simulink model "ModelCurrentState"  (R2024b)
settings: Solver=VariableStepAuto  StartTime=0.0  StopTime=StopTime  MaxStep=0.001  RelTol=1e-3
model workspace: external: MAT-File 3DModelInputs.mat (data not in the file)
undefined symbols (not defined in the file): GripStrength, KillswitchFinalValue, KillswitchInitialValue, KillswitchStepTime, LeftLowerArmLength, PlaneTilt, RightLowerArmLength, UpperTorsoLength, X, Y, Z
libraries: nesl_utility x408, sm_lib x139, matrix_library x11, simulink x1
(part 3 of 14)

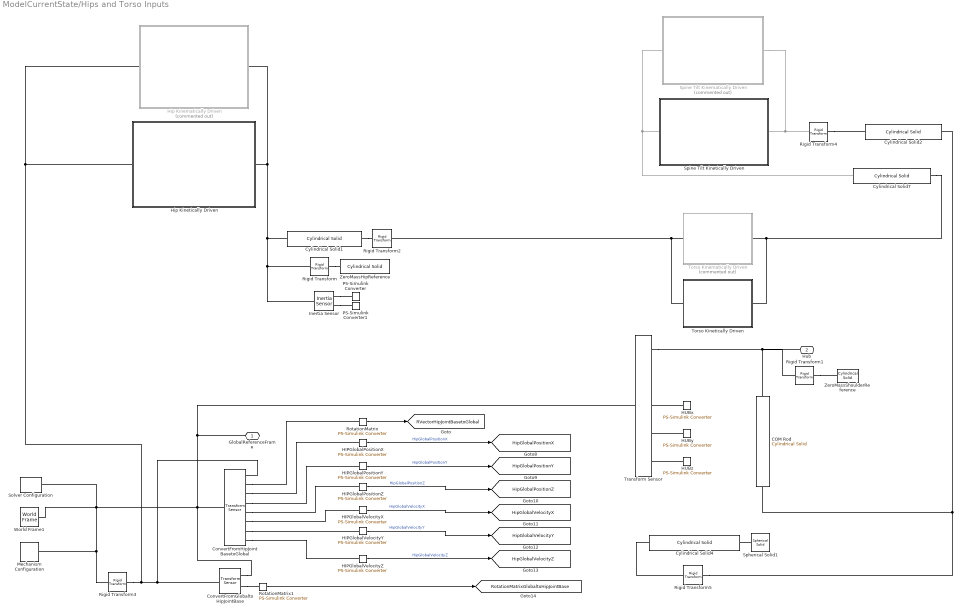
== system ModelCurrentState/Hips and Torso Inputs ==
  COM Rod : sm_lib/Body Elements/Cylindrical Solid  CylinderRadius=0.1  CylinderRadiusUnits=in  CylinderLength=2  CylinderLengthUnits=in  ExportEntireGeometry=off  InertiaType=CalculateFromGeometry  BasedOnType=Mass  Density=1000  DensityUnits=kg/m^3  Mass=0  MassUnits=kg  CenterOfMass=[0 0 0]  CenterOfMassUnits=m  MomentsOfInertia=[1 1 1]  MomentsOfInertiaUnits=kg*m^2  ProductsOfInertia=[0 0 0]  ProductsOfInertiaUnits=kg*m^2  GraphicType=FromGeometry  MarkerShape=Sphere  MarkerSize=10  GraphicVisPropType=SimpleVisualProperties  GraphicDiffuseColor=[0.5 0.5 0.5]  GraphicOpacity=1.0  GraphicSpecularColor=[0.5 0.5 0.5 1.0]  GraphicAmbientColor=[0.15 0.15 0.15 1.0]  GraphicEmissiveColor=[0.0 0.0 0.0 1.0]  GraphicShininess=75  DoExposeReferenceFrame=off  SerializedFrames=<Frames><Frame><Id>Frame1</Id><Value><Name>COM Rod Bottom</Name><Origin><Source>GeometricFeature</Source><FeatureName>top curve</FeatureName></Origin><PrimaryAxis><DefinedDirection>-X</DefinedDirection><Source>ReferenceFrame</Source><SourceDirection>-Y</SourceDirection><FeatureName></FeatureName></PrimaryAxis><SecondaryAxis><DefinedDirection>+Y</DefinedDirection><Source>ReferenceFrame</Source><SourceDirection>+Z</SourceDirection><FeatureName></FeatureName></SecondaryAxis></Value></Frame><Frame><Id>Frame2</Id><Value><Name>COM Rod Top</Name><Origin><Source>GeometricFeature</Source><FeatureName>bottom curve</FeatureName></Origin><PrimaryAxis><DefinedDirection>+X</DefinedDirection><Source>ReferenceFrame</Source><SourceDirection>+X</SourceDirection><FeatureName></FeatureName></PrimaryAxis><SecondaryAxis><DefinedDirection>+Y</DefinedDirection><Source>ReferenceFrame</Source><SourceDirection>+Z</SourceDirection><FeatureName></FeatureName></SecondaryAxis></Value></Frame></Frames>
  ConvertFromGlobaltoHipJointBase : sm_lib/Frames and Transforms/Transform Sensor  MeasurementFrame=World  RotationSequence=XYX  SenseAngle=off  SenseAxis=off  SenseQ=off  SenseR=on  SenseRotationSequence=off  SenseOmegaX=off  SenseOmegaY=off  SenseOmegaZ=off  SenseOmega=off  SenseQDot=off  SenseRDot=off  SenseRotationSequenceDot=off  SenseAlphaX=off  SenseAlphaY=off  SenseAlphaZ=off  SenseAlpha=off  SenseQDDot=off  SenseRDDot=off  SenseX=off  SenseY=off  SenseZ=off  SenseXYZ=off  SenseRad=off  SenseAzim=off  SenseDist=off  SenseInc=off  SenseXDot=off  SenseYDot=off  SenseZDot=off  SenseXYZDot=off  SenseRadDot=off  SenseAzimDot=off  SenseDistDot=off  SenseIncDot=off  SenseXDDot=off  SenseYDDot=off  SenseZDDot=off  SenseXYZDDot=off  SenseRadDDot=off  SenseAzimDDot=off  SenseDistDDot=off  SenseIncDDot=off
  ConvertFromHipJointBasetoGlobal : sm_lib/Frames and Transforms/Transform Sensor  MeasurementFrame=World  RotationSequence=XYX  SenseAngle=off  SenseAxis=off  SenseQ=off  SenseR=on  SenseRotationSequence=off  SenseOmegaX=off  SenseOmegaY=off  SenseOmegaZ=off  SenseOmega=off  SenseQDot=off  SenseRDot=off  SenseRotationSequenceDot=off  SenseAlphaX=off  SenseAlphaY=off  SenseAlphaZ=off  SenseAlpha=off  SenseQDDot=off  SenseRDDot=off  SenseX=on  SenseY=on  SenseZ=on  SenseXYZ=off  SenseRad=off  SenseAzim=off  SenseDist=off  SenseInc=off  SenseXDot=on  SenseYDot=on  SenseZDot=on  SenseXYZDot=off  SenseRadDot=off  SenseAzimDot=off  SenseDistDot=off  SenseIncDot=off  SenseXDDot=off  SenseYDDot=off  SenseZDDot=off  SenseXYZDDot=off  SenseRadDDot=off  SenseAzimDDot=off  SenseDistDDot=off  SenseIncDDot=off
  Cylindrical Solid1 : sm_lib/Body Elements/Cylindrical Solid  CylinderRadius=6  CylinderRadiusUnits=in  CylinderLength=LowerTorsoLength  CylinderLengthUnits=in  ExportEntireGeometry=off  InertiaType=CalculateFromGeometry  BasedOnType=Mass  Density=1000  DensityUnits=kg/m^3  Mass=20  MassUnits=kg  CenterOfMass=[0 0 0]  CenterOfMassUnits=m  MomentsOfInertia=[1 1 1]  MomentsOfInertiaUnits=kg*m^2  ProductsOfInertia=[0 0 0]  ProductsOfInertiaUnits=kg*m^2  GraphicType=FromGeometry  MarkerShape=Sphere  MarkerSize=10  GraphicVisPropType=SimpleVisualProperties  GraphicDiffuseColor=[0.2 0.2 0.0]  GraphicOpacity=1.0  GraphicSpecularColor=[0.5 0.5 0.5 1.0]  GraphicAmbientColor=[0.15 0.15 0.15 1.0]  GraphicEmissiveColor=[0.0 0.0 0.0 1.0]  GraphicShininess=75  DoExposeReferenceFrame=off  SerializedFrames=<Frames><Frame><Id>Frame1</Id><Value><Name>Bottom of Hips</Name><Origin><Source>GeometricFeature</Source><FeatureName>top surface</FeatureName></Origin><PrimaryAxis><DefinedDirection>-Z</DefinedDirection><Source>ReferenceFrame</Source><SourceDirection>+Z</SourceDirection><FeatureName></FeatureName></PrimaryAxis><SecondaryAxis><DefinedDirection>+X</DefinedDirection><Source>ReferenceFrame</Source><SourceDirection>+X</SourceDirection><FeatureName></FeatureName></SecondaryAxis></Value></Frame><Frame><Id>Frame2</Id><Value><Name>Top of Hips</Name><Origin><Source>GeometricFeature</Source><FeatureName>bottom surface</FeatureName></Origin><PrimaryAxis><DefinedDirection>+Z</DefinedDirection><Source>ReferenceFrame</Source><SourceDirection>+Z</SourceDirection><FeatureName></FeatureName></PrimaryAxis><SecondaryAxis><DefinedDirection>+X</DefinedDirection><Source>ReferenceFrame</Source><SourceDirection>+X</SourceDirection><FeatureName></FeatureName></SecondaryAxis></Value></Frame></Frames>
  Cylindrical Solid2 : sm_lib/Body Elements/Cylindrical Solid  CylinderRadius=6  CylinderRadiusUnits=in  CylinderLength=UpperTorsoLength*0.8  CylinderLengthUnits=in  ExportEntireGeometry=off  InertiaType=CalculateFromGeometry  BasedOnType=Mass  Density=1000  DensityUnits=kg/m^3  Mass=20*0.8  MassUnits=kg  CenterOfMass=[0 0 0]  CenterOfMassUnits=m  MomentsOfInertia=[1 1 1]  MomentsOfInertiaUnits=kg*m^2  ProductsOfInertia=[0 0 0]  ProductsOfInertiaUnits=kg*m^2  GraphicType=FromGeometry  MarkerShape=Sphere  MarkerSize=10  GraphicVisPropType=SimpleVisualProperties  GraphicDiffuseColor=[0.2 0.2 1.0]  GraphicOpacity=1.0  GraphicSpecularColor=[0.5 0.5 0.5 1.0]  GraphicAmbientColor=[0.15 0.15 0.15 1.0]  GraphicEmissiveColor=[0.0 0.0 0.0 1.0]  GraphicShininess=75  DoExposeReferenceFrame=off  SerializedFrames=<Frames><Frame><Id>Frame1</Id><Value><Name>Bottom of Torso</Name><Origin><Source>GeometricFeature</Source><FeatureName>top surface</FeatureName></Origin><PrimaryAxis><DefinedDirection>-Z</DefinedDirection><Source>ReferenceFrame</Source><SourceDirection>+Z</SourceDirection><FeatureName></FeatureName></PrimaryAxis><SecondaryAxis><DefinedDirection>+X</DefinedDirection><Source>ReferenceFrame</Source><SourceDirection>+X</SourceDirection><FeatureName></FeatureName></SecondaryAxis></Value></Frame><Frame><Id>Frame2</Id><Value><Name>Top of Torso</Name><Origin><Source>GeometricFeature</Source><FeatureName>bottom surface</FeatureName></Origin><PrimaryAxis><DefinedDirection>+Z</DefinedDirection><Source>ReferenceFrame</Source><SourceDirection>+Z</SourceDirection><FeatureName></FeatureName></PrimaryAxis><SecondaryAxis><DefinedDirection>+X</DefinedDirection><Source>ReferenceFrame</Source><SourceDirection>+X</SourceDirection><FeatureName></FeatureName></SecondaryAxis></Value></Frame></Frames>
  Cylindrical Solid4 : sm_lib/Body Elements/Cylindrical Solid  CylinderRadius=2  CylinderRadiusUnits=in  CylinderLength=10  CylinderLengthUnits=in  ExportEntireGeometry=off  InertiaType=CalculateFromGeometry  BasedOnType=Density  Density=1000  DensityUnits=kg/m^3  Mass=1  MassUnits=kg  CenterOfMass=[0 0 0]  CenterOfMassUnits=m  MomentsOfInertia=[1 1 1]  MomentsOfInertiaUnits=kg*m^2  ProductsOfInertia=[0 0 0]  ProductsOfInertiaUnits=kg*m^2  GraphicType=FromGeometry  MarkerShape=Sphere  MarkerSize=10  GraphicVisPropType=SimpleVisualProperties  GraphicDiffuseColor=[1.0 0.8 0.4]  GraphicOpacity=1.0  GraphicSpecularColor=[0.5 0.5 0.5 1.0]  GraphicAmbientColor=[0.15 0.15 0.15 1.0]  GraphicEmissiveColor=[0.0 0.0 0.0 1.0]  GraphicShininess=75  DoExposeReferenceFrame=off  SerializedFrames=<Frames><Frame><Id>Frame1</Id><Value><Name>Bottom of Neck</Name><Origin><Source>GeometricFeature</Source><FeatureName>top surface</FeatureName></Origin><PrimaryAxis><DefinedDirection>+Z</DefinedDirection><Source>ReferenceFrame</Source><SourceDirection>+Z</SourceDirection><FeatureName></FeatureName></PrimaryAxis><SecondaryAxis><DefinedDirection>+X</DefinedDirection><Source>ReferenceFrame</Source><SourceDirection>+X</SourceDirection><FeatureName></FeatureName></SecondaryAxis></Value></Frame><Frame><Id>Frame2</Id><Value><Name>Top of Neck</Name><Origin><Source>GeometricFeature</Source><FeatureName>bottom surface</FeatureName></Origin><PrimaryAxis><DefinedDirection>+Z</DefinedDirection><Source>ReferenceFrame</Source><SourceDirection>+Z</SourceDirection><FeatureName></FeatureName></PrimaryAxis><SecondaryAxis><DefinedDirection>+X</DefinedDirection><Source>ReferenceFrame</Source><SourceDirection>+X</SourceDirection><FeatureName></FeatureName></SecondaryAxis></Value></Frame></Frames>
  Cylindrical Solid7 : sm_lib/Body Elements/Cylindrical Solid  CylinderRadius=6  CylinderRadiusUnits=in  CylinderLength=UpperTorsoLength*0.2  CylinderLengthUnits=in  ExportEntireGeometry=off  InertiaType=CalculateFromGeometry  BasedOnType=Mass  Density=1000  DensityUnits=kg/m^3  Mass=20*0.2  MassUnits=kg  CenterOfMass=[0 0 0]  CenterOfMassUnits=m  MomentsOfInertia=[1 1 1]  MomentsOfInertiaUnits=kg*m^2  ProductsOfInertia=[0 0 0]  ProductsOfInertiaUnits=kg*m^2  GraphicType=FromGeometry  MarkerShape=Sphere  MarkerSize=10  GraphicVisPropType=SimpleVisualProperties  GraphicDiffuseColor=[0.2 0.2 1.0]  GraphicOpacity=1.0  GraphicSpecularColor=[0.5 0.5 0.5 1.0]  GraphicAmbientColor=[0.15 0.15 0.15 1.0]  GraphicEmissiveColor=[0.0 0.0 0.0 1.0]  GraphicShininess=75  DoExposeReferenceFrame=off  SerializedFrames=<Frames><Frame><Id>Frame1</Id><Value><Name>Bottom of Torso</Name><Origin><Source>GeometricFeature</Source><FeatureName>top surface</FeatureName></Origin><PrimaryAxis><DefinedDirection>-Z</DefinedDirection><Source>ReferenceFrame</Source><SourceDirection>+Z</SourceDirection><FeatureName></FeatureName></PrimaryAxis><SecondaryAxis><DefinedDirection>+X</DefinedDirection><Source>ReferenceFrame</Source><SourceDirection>+X</SourceDirection><FeatureName></FeatureName></SecondaryAxis></Value></Frame><Frame><Id>Frame2</Id><Value><Name>Top of Torso</Name><Origin><Source>GeometricFeature</Source><FeatureName>bottom surface</FeatureName></Origin><PrimaryAxis><DefinedDirection>+Z</DefinedDirection><Source>ReferenceFrame</Source><SourceDirection>+Z</SourceDirection><FeatureName></FeatureName></PrimaryAxis><SecondaryAxis><DefinedDirection>+X</DefinedDirection><Source>ReferenceFrame</Source><SourceDirection>+X</SourceDirection><FeatureName></FeatureName></SecondaryAxis></Value></Frame></Frames>
  HIPGlobalPositionX : nesl_utility/PS-Simulink Converter  PhysicalDomain=network_engine_domain  SubClassName=ps_output  LeftPortType=input  RightPortType=output  PseudoPeriodic=off  Frequencies=[]  VectorFormat=inherit  Unit=m  AffineConversion=off
  HIPGlobalPositionY : nesl_utility/PS-Simulink Converter  PhysicalDomain=network_engine_domain  SubClassName=ps_output  LeftPortType=input  RightPortType=output  PseudoPeriodic=off  Frequencies=[]  VectorFormat=inherit  Unit=m  AffineConversion=off
  HIPGlobalPositionZ : nesl_utility/PS-Simulink Converter  PhysicalDomain=network_engine_domain  SubClassName=ps_output  LeftPortType=input  RightPortType=output  PseudoPeriodic=off  Frequencies=[]  VectorFormat=inherit  Unit=m  AffineConversion=off
  HIPGlobalVelocityX : nesl_utility/PS-Simulink Converter  PhysicalDomain=network_engine_domain  SubClassName=ps_output  LeftPortType=input  RightPortType=output  PseudoPeriodic=off  Frequencies=[]  VectorFormat=1-D array  Unit=m/s  AffineConversion=off
  HIPGlobalVelocityY : nesl_utility/PS-Simulink Converter  PhysicalDomain=network_engine_domain  SubClassName=ps_output  LeftPortType=input  RightPortType=output  PseudoPeriodic=off  Frequencies=[]  VectorFormat=1-D array  Unit=m/s  AffineConversion=off
  HIPGlobalVelocityZ : nesl_utility/PS-Simulink Converter  PhysicalDomain=network_engine_domain  SubClassName=ps_output  LeftPortType=input  RightPortType=output  PseudoPeriodic=off  Frequencies=[]  VectorFormat=1-D array  Unit=m/s  AffineConversion=off
  HUBx : nesl_utility/PS-Simulink Converter  PhysicalDomain=network_engine_domain  SubClassName=ps_output  LeftPortType=input  RightPortType=output  PseudoPeriodic=off  Frequencies=[]  VectorFormat=1-D array  Unit=inherit  AffineConversion=off
  HUBy : nesl_utility/PS-Simulink Converter  PhysicalDomain=network_engine_domain  SubClassName=ps_output  LeftPortType=input  RightPortType=output  PseudoPeriodic=off  Frequencies=[]  VectorFormat=1-D array  Unit=inherit  AffineConversion=off
  HUBz : nesl_utility/PS-Simulink Converter  PhysicalDomain=network_engine_domain  SubClassName=ps_output  LeftPortType=input  RightPortType=output  PseudoPeriodic=off  Frequencies=[]  VectorFormat=1-D array  Unit=inherit  AffineConversion=off
  Hip Kinematically Driven : Subsystem  Commented=on
  Hip Kinetically Driven : Subsystem
  Inertia Sensor : sm_lib/Body Elements/Inertia Sensor  SensorExtent=Mechanism  SpanWeldJoints=off  ExcludeGroundedBodies=off  MeasurementFrame=World  SenseMass=on  SenseCenterOfMass=on  SenseInertiaMatrix=off  SenseCenteredInertiaMatrix=off  SensePrincipalInertiaMatrix=off  SenseRotationMatrix=off  GraphicType=None  PrincipalInertiaFrameSize=20  GraphicVisPropType=SimpleVisualProperties  GraphicDiffuseColor=[0.5 0.5 0.5]  GraphicOpacity=1  GraphicSpecularColor=[0.5 0.5 0.5 1.0]  GraphicAmbientColor=[0.15 0.15 0.15 1.0]  GraphicEmissiveColor=[0.0 0.0 0.0 1.0]  GraphicShininess=75
  Mechanism Configuration : sm_lib/Utilities/Mechanism Configuration  UniformGravity=Constant  GravityVector=[0 0 -9.80665]  GravityVectorUnits=m/s^2  LinearizationDelta=0.001  JointModeTransitionNonlinearIterations=2
  PS-Simulink Converter : nesl_utility/PS-Simulink Converter  PhysicalDomain=network_engine_domain  SubClassName=ps_output  LeftPortType=input  RightPortType=output  PseudoPeriodic=off  Frequencies=[]  VectorFormat=1-D array  Unit=inherit  AffineConversion=off
  PS-Simulink Converter1 : nesl_utility/PS-Simulink Converter  PhysicalDomain=network_engine_domain  SubClassName=ps_output  LeftPortType=input  RightPortType=output  PseudoPeriodic=off  Frequencies=[]  VectorFormat=1-D array  Unit=inherit  AffineConversion=off
  Rigid Transform : sm_lib/Frames and Transforms/Rigid Transform  RotationMethod=RotationSequence  FollAlignAxisA=+X  BaseAlignAxisA=+Y  FollAlignAxisB=+Y  BaseAlignAxisB=+Z  RotationStandardAxis=+Z  RotationAngle=0.0  RotationAngleUnits=deg  RotationArbitraryAxis=[0 0 1]  RotationSequenceAxes=BaseAxes  RotationSequence=XYX  RotationSequenceAngles=[0 90 0]  RotationSequenceAnglesUnits=deg  RotationMatrix=[1 0 0; 0 1 0; 0 0 1]  Quaternion=[1 0 0 0]  TranslationMethod=None  TranslationCartesianOffset=[0 0 0]  TranslationCartesianOffsetUnits=m  TranslationStandardAxis=+Z  TranslationStandardOffset=0  TranslationStandardOffsetUnits=m  TranslationROffset=0  TranslationROffsetUnits=m  TranslationThetaOffset=0  TranslationThetaOffsetUnits=deg  TranslationZOffset=0  TranslationZOffsetUnits=m
  Rigid Transform1 : sm_lib/Frames and Transforms/Rigid Transform  RotationMethod=RotationSequence  FollAlignAxisA=+X  BaseAlignAxisA=+Y  FollAlignAxisB=+Y  BaseAlignAxisB=+Z  RotationStandardAxis=+Z  RotationAngle=0.0  RotationAngleUnits=deg  RotationArbitraryAxis=[0 0 1]  RotationSequenceAxes=BaseAxes  RotationSequence=XYX  RotationSequenceAngles=[0 0 0]  RotationSequenceAnglesUnits=deg  RotationMatrix=[1 0 0; 0 1 0; 0 0 1]  Quaternion=[1 0 0 0]  TranslationMethod=None  TranslationCartesianOffset=[0 0 0]  TranslationCartesianOffsetUnits=m  TranslationStandardAxis=+Z  TranslationStandardOffset=0  TranslationStandardOffsetUnits=m  TranslationROffset=0  TranslationROffsetUnits=m  TranslationThetaOffset=0  TranslationThetaOffsetUnits=deg  TranslationZOffset=0  TranslationZOffsetUnits=m
  Rigid Transform2 : sm_lib/Frames and Transforms/Rigid Transform  RotationMethod=RotationSequence  FollAlignAxisA=+X  BaseAlignAxisA=+Y  FollAlignAxisB=+Y  BaseAlignAxisB=+Z  RotationStandardAxis=+Z  RotationAngle=0.0  RotationAngleUnits=deg  RotationArbitraryAxis=[0 0 1]  RotationSequenceAxes=BaseAxes  RotationSequence=XYZ  RotationSequenceAngles=[180 0 0]  RotationSequenceAnglesUnits=deg  RotationMatrix=[1 0 0; 0 1 0; 0 0 1]  Quaternion=[1 0 0 0]  TranslationMethod=None  TranslationCartesianOffset=[0 0 0]  TranslationCartesianOffsetUnits=m  TranslationStandardAxis=+Z  TranslationStandardOffset=0  TranslationStandardOffsetUnits=m  TranslationROffset=0  TranslationROffsetUnits=m  TranslationThetaOffset=0  TranslationThetaOffsetUnits=deg  TranslationZOffset=0  TranslationZOffsetUnits=m
  Rigid Transform3 : sm_lib/Frames and Transforms/Rigid Transform  RotationMethod=RotationSequence  FollAlignAxisA=+X  BaseAlignAxisA=+Y  FollAlignAxisB=+Y  BaseAlignAxisB=+Z  RotationStandardAxis=+Z  RotationAngle=0.0  RotationAngleUnits=deg  RotationArbitraryAxis=[0 0 1]  RotationSequenceAxes=BaseAxes  RotationSequence=ZXZ  RotationSequenceAngles=[0 PlaneTilt 0]  RotationSequenceAnglesUnits=deg  RotationMatrix=[1 0 0; 0 1 0; 0 0 1]  Quaternion=[1 0 0 0]  TranslationMethod=None  TranslationCartesianOffset=[0 0 0]  TranslationCartesianOffsetUnits=m  TranslationStandardAxis=+Z  TranslationStandardOffset=0  TranslationStandardOffsetUnits=m  TranslationROffset=0  TranslationROffsetUnits=m  TranslationThetaOffset=0  TranslationThetaOffsetUnits=deg  TranslationZOffset=0  TranslationZOffsetUnits=m
  Rigid Transform4 : sm_lib/Frames and Transforms/Rigid Transform  RotationMethod=RotationSequence  FollAlignAxisA=+X  BaseAlignAxisA=+Y  FollAlignAxisB=+Y  BaseAlignAxisB=+Z  RotationStandardAxis=+Z  RotationAngle=0  RotationAngleUnits=deg  RotationArbitraryAxis=[0 0 1]  RotationSequenceAxes=FollowerAxes  RotationSequence=XYZ  RotationSequenceAngles=[180 0 0]  RotationSequenceAnglesUnits=deg  RotationMatrix=[1 0 0;0 1 0;0 0 1]  Quaternion=[1 0 0 0]  TranslationMethod=None  TranslationCartesianOffset=[0 0 0]  TranslationCartesianOffsetUnits=m  TranslationStandardAxis=+Z  TranslationStandardOffset=0  TranslationStandardOffsetUnits=m  TranslationROffset=0  TranslationROffsetUnits=m  TranslationThetaOffset=0  TranslationThetaOffsetUnits=deg  TranslationZOffset=0  TranslationZOffsetUnits=m
  Rigid Transform5 : sm_lib/Frames and Transforms/Rigid Transform  RotationMethod=RotationSequence  FollAlignAxisA=+X  BaseAlignAxisA=+Y  FollAlignAxisB=+Y  BaseAlignAxisB=+Z  RotationStandardAxis=+Z  RotationAngle=0.0  RotationAngleUnits=deg  RotationArbitraryAxis=[0 0 1]  RotationSequenceAxes=BaseAxes  RotationSequence=XYX  RotationSequenceAngles=[0 0 0]  RotationSequenceAnglesUnits=deg  RotationMatrix=[1 0 0; 0 1 0; 0 0 1]  Quaternion=[1 0 0 0]  TranslationMethod=None  TranslationCartesianOffset=[0 0 0]  TranslationCartesianOffsetUnits=m  TranslationStandardAxis=+Z  TranslationStandardOffset=0  TranslationStandardOffsetUnits=m  TranslationROffset=0  TranslationROffsetUnits=m  TranslationThetaOffset=0  TranslationThetaOffsetUnits=deg  TranslationZOffset=0  TranslationZOffsetUnits=m
  RotationMatrix : nesl_utility/PS-Simulink Converter  PhysicalDomain=network_engine_domain  SubClassName=ps_output  LeftPortType=input  RightPortType=output  PseudoPeriodic=off  Frequencies=[]  VectorFormat=1-D array  Unit=inherit  AffineConversion=off
  RotationMatrix1 : nesl_utility/PS-Simulink Converter  PhysicalDomain=network_engine_domain  SubClassName=ps_output  LeftPortType=input  RightPortType=output  PseudoPeriodic=off  Frequencies=[]  VectorFormat=1-D array  Unit=inherit  AffineConversion=off
  Solver Configuration : nesl_utility/Solver Configuration  PhysicalDomain=network_engine_domain  SubClassName=solver  LeftPortType=input  RightPortType=generic  Tones=[]  Harmonics=[]  SimulateNoise=off  Profile=off  UseLocalSampling=off  EnableSwitchedLinearOptims=on  FrequencyDomain=off  UseCCode=off  RelTol=0.001  AbsTol=0.001  MinStep=1e-09  ToWorkspace=off  RevertToSquareIcSolve=off  NumHomotopyIterations=100  PhasorMode=off  PhasorModeNumHarmonics=1  ConsistencySolver=NEWTON_XTOL_AFTER_FTOL  IndexReductionMethod=DerivativeReplacement  DoDC=off  ResidualTolerance=1e-09  ConsistencyTolSource=GLOBAL  ConsistencyAbsTol=0.001  ConsistencyRelTol=0.001  ConsistencyTolFactor=0.001  UseLocalSolver=off  LocalSolverChoice=NE_BACKWARD_EULER_ADVANCER  ResolveIndetEquations=on  FunctionEvalNumThread=1  LocalSolverSampleTime=0.001  DoFixedCost=off  MaxNonlinIter=3  MaxModeIter=2  ComputeImpulses=off  ImpulseIterations=2  LinearAlgebra=auto  LinearAlgebraNumThread=0  EquationFormulation=NE_TIME_EF  DelaysMemoryBudget=1024  AutomaticFiltering=on  FilteringTimeConstant=0.001  PartitionStorageMethod=AS_NEEDED  PartitionMemoryBudget=1024  PartitionMethod=ROBUST  MultibodyUseLocalSolver=off  MultibodyLocalSolverChoice=ODE1  MultibodyLocalSolverSampleTime=0.001
  Spherical Solid1 : sm_lib/Body Elements/Spherical Solid  SphereRadius=5  SphereRadiusUnits=in  ExportEntireGeometry=off  InertiaType=CalculateFromGeometry  BasedOnType=Mass  Density=1000  DensityUnits=kg/m^3  Mass=11  MassUnits=lbm  CenterOfMass=[0 0 0]  CenterOfMassUnits=m  MomentsOfInertia=[1 1 1]  MomentsOfInertiaUnits=kg*m^2  ProductsOfInertia=[0 0 0]  ProductsOfInertiaUnits=kg*m^2  GraphicType=FromGeometry  MarkerShape=Sphere  MarkerSize=10  GraphicVisPropType=SimpleVisualProperties  GraphicDiffuseColor=[1.0 0.8 0.4]  GraphicOpacity=1.0  GraphicSpecularColor=[0.5 0.5 0.5 1.0]  GraphicAmbientColor=[0.15 0.15 0.15 1.0]  GraphicEmissiveColor=[0.0 0.0 0.0 1.0]  GraphicShininess=75  DoExposeReferenceFrame=on  SerializedFrames=<Frames/>
  Spine Tilt Kinematically Driven : Subsystem  Commented=on
  Spine Tilt Kinetically Driven : Subsystem
  Torso Kinematically Driven : Subsystem  Commented=on
  Torso Kinetically Driven : Subsystem
  Transform Sensor : sm_lib/Frames and Transforms/Transform Sensor  MeasurementFrame=World  RotationSequence=XYX  SenseAngle=off  SenseAxis=off  SenseQ=off  SenseR=on  SenseRotationSequence=off  SenseOmegaX=off  SenseOmegaY=off  SenseOmegaZ=off  SenseOmega=off  SenseQDot=off  SenseRDot=off  SenseRotationSequenceDot=off  SenseAlphaX=off  SenseAlphaY=off  SenseAlphaZ=off  SenseAlpha=off  SenseQDDot=off  SenseRDDot=off  SenseX=on  SenseY=on  SenseZ=on  SenseXYZ=off  SenseRad=off  SenseAzim=off  SenseDist=off  SenseInc=off  SenseXDot=off  SenseYDot=off  SenseZDot=off  SenseXYZDot=off  SenseRadDot=off  SenseAzimDot=off  SenseDistDot=off  SenseIncDot=off  SenseXDDot=off  SenseYDDot=off  SenseZDDot=off  SenseXYZDDot=off  SenseRadDDot=off  SenseAzimDDot=off  SenseDistDDot=off  SenseIncDDot=off
  World Frame1 : sm_lib/Frames and Transforms/World Frame
  ZeroMassHipReference : sm_lib/Body Elements/Cylindrical Solid  CylinderRadius=4  CylinderRadiusUnits=in  CylinderLength=12  CylinderLengthUnits=in  ExportEntireGeometry=off  InertiaType=CalculateFromGeometry  BasedOnType=Mass  Density=1000  DensityUnits=kg/m^3  Mass=0  MassUnits=kg  CenterOfMass=[0 0 0]  CenterOfMassUnits=m  MomentsOfInertia=[1 1 1]  MomentsOfInertiaUnits=kg*m^2  ProductsOfInertia=[0 0 0]  ProductsOfInertiaUnits=kg*m^2  GraphicType=FromGeometry  MarkerShape=Sphere  MarkerSize=10  GraphicVisPropType=SimpleVisualProperties  GraphicDiffuseColor=[0.2 0.2 0.0]  GraphicOpacity=1.0  GraphicSpecularColor=[0.5 0.5 0.5 1.0]  GraphicAmbientColor=[0.15 0.15 0.15 1.0]  GraphicEmissiveColor=[0.0 0.0 0.0 1.0]  GraphicShininess=75  DoExposeReferenceFrame=on  SerializedFrames=<Frames/>
  ZeroMassShoulderReference : sm_lib/Body Elements/Cylindrical Solid  CylinderRadius=3  CylinderRadiusUnits=in  CylinderLength=12  CylinderLengthUnits=in  ExportEntireGeometry=off  InertiaType=CalculateFromGeometry  BasedOnType=Mass  Density=1000  DensityUnits=kg/m^3  Mass=0  MassUnits=kg  CenterOfMass=[0 0 0]  CenterOfMassUnits=m  MomentsOfInertia=[1 1 1]  MomentsOfInertiaUnits=kg*m^2  ProductsOfInertia=[0 0 0]  ProductsOfInertiaUnits=kg*m^2  GraphicType=FromGeometry  MarkerShape=Sphere  MarkerSize=10  GraphicVisPropType=SimpleVisualProperties  GraphicDiffuseColor=[0.07451 0.6235 1]  GraphicOpacity=1.0  GraphicSpecularColor=[0.5 0.5 0.5 1.0]  GraphicAmbientColor=[0.15 0.15 0.15 1.0]  GraphicEmissiveColor=[0.0 0.0 0.0 1.0]  GraphicShininess=75  DoExposeReferenceFrame=on  SerializedFrames=<Frames/>
  GlobalReferenceFrame : PMIOPort  Side=Right
  Hub : PMIOPort  Port=2  Side=Left
  tag scope: HipGlobalPositionX=global, HipGlobalPositionY=global, HipGlobalPositionZ=global, HipGlobalVelocityX=global, HipGlobalVelocityY=global, HipGlobalVelocityZ=global, RVectorHipJointBasetoGlobal=global, RotationMatrixGlobaltoHipJointBase=global
  wires:
  RotationMatrix1/1 -> [RotationMatrixGlobaltoHipJointBase]
  HIPGlobalVelocityZ/1 -> [HipGlobalVelocityZ]  "HipGlobalVelocityZ"
  HIPGlobalVelocityY/1 -> [HipGlobalVelocityY]  "HipGlobalVelocityY"
  HIPGlobalVelocityX/1 -> [HipGlobalVelocityX]  "HipGlobalVelocityX"
  HIPGlobalPositionY/1 -> [HipGlobalPositionY]  "HipGlobalPositionY"
  HIPGlobalPositionX/1 -> [HipGlobalPositionX]  "HipGlobalPositionX"
  HIPGlobalPositionZ/1 -> [HipGlobalPositionZ]  "HipGlobalPositionZ"
  RotationMatrix/1 -> [RVectorHipJointBasetoGlobal]
  connections:
  HUBy/LConn1 -- Transform Sensor/RConn4
  Spine Tilt Kinematically Driven/LConn1 -- Cylindrical Solid7/RConn1 -- Spine Tilt Kinetically Driven/LConn1
  COM Rod/RConn1 -- Transform Sensor/RConn1 -- Rigid Transform1/RConn1 -- Hub/RConn1
  Rigid Transform5/LConn1 -- COM Rod/LConn1 -- Cylindrical Solid2/RConn1
  Rigid Transform1/LConn1 -- ZeroMassShoulderReference/RConn1
  HUBx/LConn1 -- Transform Sensor/RConn3
  Spherical Solid1/RConn1 -- Cylindrical Solid4/RConn1
  Rigid Transform5/RConn1 -- Cylindrical Solid4/LConn1
  HUBz/LConn1 -- Transform Sensor/RConn5
  Rigid Transform4/RConn1 -- Cylindrical Solid2/LConn1
  Transform Sensor/LConn1 -- GlobalReferenceFrame/RConn1 -- ConvertFromHipJointBasetoGlobal/LConn1 -- ConvertFromGlobaltoHipJointBase/RConn1 -- Solver Configuration/RConn1 -- Mechanism Configuration/RConn1 -- Rigid Transform3/LConn1 -- World Frame1/RConn1
  ConvertFromGlobaltoHipJointBase/RConn2 -- RotationMatrix1/LConn1
  ConvertFromHipJointBasetoGlobal/RConn8 -- HIPGlobalVelocityZ/LConn1
  ConvertFromHipJointBasetoGlobal/RConn7 -- HIPGlobalVelocityY/LConn1
  ConvertFromHipJointBasetoGlobal/RConn6 -- HIPGlobalVelocityX/LConn1
  ConvertFromHipJointBasetoGlobal/RConn3 -- HIPGlobalPositionX/LConn1
  Rigid Transform/LConn1 -- ZeroMassHipReference/RConn1
  ConvertFromHipJointBasetoGlobal/RConn4 -- HIPGlobalPositionY/LConn1
  Inertia Sensor/RConn2 -- PS-Simulink Converter1/LConn1
  Inertia Sensor/RConn1 -- PS-Simulink Converter/LConn1
  Cylindrical Solid1/RConn1 -- Rigid Transform2/LConn1
  ConvertFromHipJointBasetoGlobal/RConn2 -- RotationMatrix/LConn1
  ConvertFromHipJointBasetoGlobal/RConn5 -- HIPGlobalPositionZ/LConn1
  Cylindrical Solid7/LConn1 -- Torso Kinetically Driven/RConn1 -- Torso Kinematically Driven/RConn1
  Cylindrical Solid1/LConn1 -- Inertia Sensor/LConn1 -- Rigid Transform/RConn1 -- Hip Kinetically Driven/RConn1 -- Hip Kinematically Driven/RConn1
  Rigid Transform3/RConn1 -- ConvertFromGlobaltoHipJointBase/LConn1 -- ConvertFromHipJointBasetoGlobal/RConn1 -- Hip Kinetically Driven/LConn1 -- Hip Kinematically Driven/LConn1
  Spine Tilt Kinematically Driven/RConn1 -- Rigid Transform4/LConn1 -- Spine Tilt Kinetically Driven/RConn1
  Torso Kinetically Driven/LConn1 -- Rigid Transform2/RConn1 -- Torso Kinematically Driven/LConn1

== system ModelCurrentState/LE Input Function ==
  Left Elbow Input Torque : MATLAB Function  TreatAsAtomicUnit=on  SystemSampleTime=0
  tag scope: FcnOutLEAcceleration=global, FcnOutLEPosition=global, FcnOutLETorque=global, FcnOutLEVelocity=global
  wires:
  [LEPosition] -> Left Elbow Input Torque/3(LEPosition)
  [Time] -> Left Elbow Input Torque/1(Time)
  [LEVelocity] -> Left Elbow Input Torque/4(LEVelocity)
  Left Elbow Input Torque/2(LEPositionInput) -> [FcnOutLEPosition]
  Left Elbow Input Torque/1(JointTorqueLE) -> [FcnOutLETorque]  "LETorqueInput"
  Left Elbow Input Torque/3(LEVelocityInput) -> [FcnOutLEVelocity]
  [Killswitch] -> Left Elbow Input Torque/2(Killswitch)
  Left Elbow Input Torque/4(LEAccelerationInput) -> [FcnOutLEAcceleration]

== system ModelCurrentState/LF Input Function ==
  LF Input Torque : MATLAB Function  TreatAsAtomicUnit=on  SystemSampleTime=0
  tag scope: FcnOutLFAcceleration=global, FcnOutLFPosition=global, FcnOutLFTorque=global, FcnOutLFVelocity=global
  wires:
  LF Input Torque/3(LFVelocityInput) -> [FcnOutLFVelocity]
  LF Input Torque/2(LFPositionInput) -> [FcnOutLFPosition]
  [Killswitch] -> LF Input Torque/2(Killswitch)
  [LFPosition] -> LF Input Torque/3(LFPosition)
  [LFVelocity] -> LF Input Torque/4(LFVelocity)
  [Time] -> LF Input Torque/1(Time)
  LF Input Torque/1(JointTorqueLF) -> [FcnOutLFTorque]  "LFTorqueInput"
  LF Input Torque/4(LFAccelerationInput) -> [FcnOutLFAcceleration]

== system ModelCurrentState/LS Input Function ==
  Left Shoulder Torque Output : MATLAB Function  TreatAsAtomicUnit=on  SystemSampleTime=0
  tag scope: FcnOutLSAccelerationX=global, FcnOutLSAccelerationY=global, FcnOutLSAccelerationZ=global, FcnOutLSPositionX=global, FcnOutLSPositionY=global, FcnOutLSPositionZ=global, FcnOutLSTorqueX=global, FcnOutLSTorqueY=global, FcnOutLSTorqueZ=global, FcnOutLSVelocityX=global, FcnOutLSVelocityY=global, FcnOutLSVelocityZ=global
  wires:
  [Killswitch] -> Left Shoulder Torque Output/2(Killswitch)
  Left Shoulder Torque Output/1(JointTorqueLSX) -> [FcnOutLSTorqueX]  "LSTorqueXInput"
  Left Shoulder Torque Output/4(LSPositionInputX) -> [FcnOutLSPositionX]  "LSPositionX"
  Left Shoulder Torque Output/7(LSVelocityInputX) -> [FcnOutLSVelocityX]  "LSVelocityX"
  [Time] -> Left Shoulder Torque Output/1(Time)
  Left Shoulder Torque Output/12(LSAccelerationInputZ) -> [FcnOutLSAccelerationZ]  "LSAccelerationZ"
  Left Shoulder Torque Output/2(JointTorqueLSY) -> [FcnOutLSTorqueY]  "LSTorqueYInput"
  Left Shoulder Torque Output/8(LSVelocityInputY) -> [FcnOutLSVelocityY]  "LSVelocityY"
  Left Shoulder Torque Output/11(LSAccelerationInputY) -> [FcnOutLSAccelerationY]  "LSAccelerationY"
  Left Shoulder Torque Output/5(LSPositionInputY) -> [FcnOutLSPositionY]  "LSPositionY"
  Left Shoulder Torque Output/10(LSAccelerationInputX) -> [FcnOutLSAccelerationX]  "LSAccelerationX"
  Left Shoulder Torque Output/9(LSVelocityInputZ) -> [FcnOutLSVelocityZ]  "LSVelocityZ"
  Left Shoulder Torque Output/3(JointTorqueLSZ) -> [FcnOutLSTorqueZ]  "LSTorqueZInput"
  Left Shoulder Torque Output/6(LSPositionInputZ) -> [FcnOutLSPositionZ]  "LSPositionZ"
  [LSPositionX] -> Left Shoulder Torque Output/3(LSPositionX)
  [LSPositionY] -> Left Shoulder Torque Output/4(LSPositionY)
  [LSPositionZ] -> Left Shoulder Torque Output/5(LSPositionZ)
  [LSVelocityX] -> Left Shoulder Torque Output/6(LSVelocityX)
  [LSVelocityY] -> Left Shoulder Torque Output/7(LSVelocityY)
  [LSVelocityZ] -> Left Shoulder Torque Output/8(LSVelocityZ)

== system ModelCurrentState/LScap Input Function ==
  LScap Torque : MATLAB Function  TreatAsAtomicUnit=on  SystemSampleTime=0
  tag scope: FcnOutLScapAccelerationX=global, FcnOutLScapAccelerationY=global, FcnOutLScapPositionX=global, FcnOutLScapPositionY=global, FcnOutLScapTorqueX=global, FcnOutLScapTorqueY=global, FcnOutLScapVelocityX=global, FcnOutLScapVelocityY=global
  wires:
  LScap Torque/1(JointTorqueLScapX) -> [FcnOutLScapTorqueX]  "LScapTorqueXInput"
  LScap Torque/6(LScapVelocityInputY) -> [FcnOutLScapVelocityY]
  [LScapPositionY] -> LScap Torque/4(LScapPositionY)
  [LScapPositionX] -> LScap Torque/3(LScapPositionX)
  LScap Torque/7(LScapAccelerationInputX) -> [FcnOutLScapAccelerationX]
  LScap Torque/2(JointTorqueLScapY) -> [FcnOutLScapTorqueY]  "LScapTorqueYInput"
  LScap Torque/8(LScapAccelerationInputY) -> [FcnOutLScapAccelerationY]
  [Killswitch] -> LScap Torque/2(Killswitch)
  [Time] -> LScap Torque/1(Time)
  LScap Torque/3(LScapPositionInputX) -> [FcnOutLScapPositionX]
  LScap Torque/4(LScapPositionInputY) -> [FcnOutLScapPositionY]
  LScap Torque/5(LScapVelocityInputX) -> [FcnOutLScapVelocityX]
  [LScapVelocityX] -> LScap Torque/5(LScapVelocityX)
  [LScapVelocityY] -> LScap Torque/6(LScapVelocityY)

== system ModelCurrentState/LW Input Function ==
  Left Wrist Torque : MATLAB Function  TreatAsAtomicUnit=on  SystemSampleTime=0
  LWJointTorqueInputGlobal : Outport  PortDimensions=3
  LWConstraintTorque : Outport  Port=2  PortDimensions=3
  tag scope: FcnOutLWAccelerationX=global, FcnOutLWAccelerationY=global, FcnOutLWPositionX=global, FcnOutLWPositionY=global, FcnOutLWTorqueX=global, FcnOutLWTorqueY=global, FcnOutLWVelocityX=global, FcnOutLWVelocityY=global, LWConstraintTorque=global, LWJointTorqueInputGlobal=global
  wires:
  Left Wrist Torque/1(JointTorqueLWX) -> [FcnOutLWTorqueX]  "LWTorqueXInput"
  [Time] -> Left Wrist Torque/1(Time)
  Left Wrist Torque/5(LWVelocityInputX) -> [FcnOutLWVelocityX]
  [Killswitch] -> Left Wrist Torque/2(Killswitch)
  Left Wrist Torque/2(JointTorqueLWY) -> [FcnOutLWTorqueY]  "LWTorqueYInput"
  Left Wrist Torque/8(LWAccelerationInputY) -> [FcnOutLWAccelerationY]
  Left Wrist Torque/7(LWAccelerationInputX) -> [FcnOutLWAccelerationX]
  Left Wrist Torque/6(LWVelocityInputY) -> [FcnOutLWVelocityY]
  Left Wrist Torque/4(LWPositionInputY) -> [FcnOutLWPositionY]  "LWPositionInputY"
  Left Wrist Torque/3(LWPositionInputX) -> [FcnOutLWPositionX]  "LWPositionInputX"
  [LWPositionX] -> Left Wrist Torque/3(LWPositionX)
  [LWPositionY] -> Left Wrist Torque/4(LWPositionY)
  [LWVelocityX] -> Left Wrist Torque/5(LWVelocityX)
  [LWVelocityY] -> Left Wrist Torque/6(LWVelocityY)
  [LWLocaltoGlobalR] -> Left Wrist Torque/7(LWLocaltoGlobalR)
  [LWTorqueGlobal] -> Left Wrist Torque/8(LWTorqueGlobal)
  Left Wrist Torque/10(LWConstraintTorque) -> LWConstraintTorque/1, [LWConstraintTorque]  "LWConstraintTorque"
  Left Wrist Torque/9(LWJointTorqueInputGlobal) -> LWJointTorqueInputGlobal/1, [LWJointTorqueInputGlobal]  "LWJointTorqueInputGlobal"

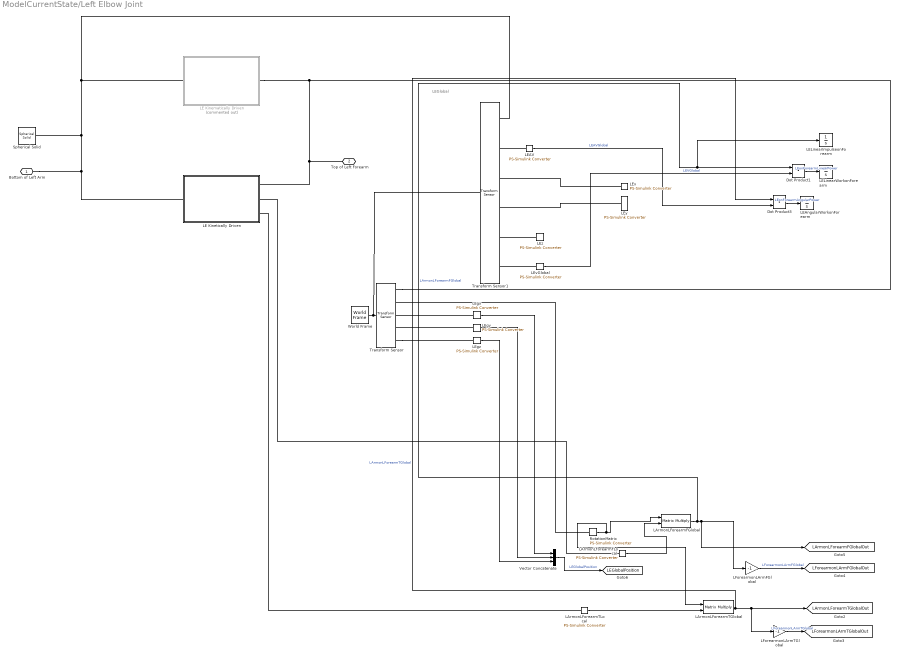
== system ModelCurrentState/Left Elbow Joint ==
  note: LEGlobal
  Dot Product1 : DotProduct  OutDataTypeStr=Inherit: Inherit via internal rule
  Dot Product3 : DotProduct  OutDataTypeStr=Inherit: Inherit via internal rule
  LArmonLForearmFGlobal : Product  Multiplication=Matrix(*)
  LArmonLForearmFLocal : nesl_utility/PS-Simulink Converter  PhysicalDomain=network_engine_domain  SubClassName=ps_output  LeftPortType=input  RightPortType=output  PseudoPeriodic=off  Frequencies=[]  VectorFormat=1-D array  Unit=inherit  AffineConversion=off
  LArmonLForearmTGlobal : Product  Multiplication=Matrix(*)
  LArmonLForearmTLocal : nesl_utility/PS-Simulink Converter  PhysicalDomain=network_engine_domain  SubClassName=ps_output  LeftPortType=input  RightPortType=output  PseudoPeriodic=off  Frequencies=[]  VectorFormat=1-D array  Unit=inherit  AffineConversion=off
  LE Kinematically Driven : Subsystem  Commented=on
  LE Kinetically Driven : Subsystem
  LEAV : nesl_utility/PS-Simulink Converter  PhysicalDomain=network_engine_domain  SubClassName=ps_output  LeftPortType=input  RightPortType=output  PseudoPeriodic=off  Frequencies=[]  VectorFormat=1-D array  Unit=inherit  AffineConversion=off
  LEAngularWorkonForearm : Integrator
  LELinearImpulseonForearm : Integrator
  LELinearWorkonForearm : Integrator
  LEgx : nesl_utility/PS-Simulink Converter  PhysicalDomain=network_engine_domain  SubClassName=ps_output  LeftPortType=input  RightPortType=output  PseudoPeriodic=off  Frequencies=[]  VectorFormat=1-D array  Unit=inherit  AffineConversion=off
  LEgy : nesl_utility/PS-Simulink Converter  PhysicalDomain=network_engine_domain  SubClassName=ps_output  LeftPortType=input  RightPortType=output  PseudoPeriodic=off  Frequencies=[]  VectorFormat=1-D array  Unit=inherit  AffineConversion=off
  LEgz : nesl_utility/PS-Simulink Converter  PhysicalDomain=network_engine_domain  SubClassName=ps_output  LeftPortType=input  RightPortType=output  PseudoPeriodic=off  Frequencies=[]  VectorFormat=1-D array  Unit=inherit  AffineConversion=off
  LEvGlobal : nesl_utility/PS-Simulink Converter  PhysicalDomain=network_engine_domain  SubClassName=ps_output  LeftPortType=input  RightPortType=output  PseudoPeriodic=off  Frequencies=[]  VectorFormat=1-D array  Unit=inherit  AffineConversion=off
  LEx : nesl_utility/PS-Simulink Converter  PhysicalDomain=network_engine_domain  SubClassName=ps_output  LeftPortType=input  RightPortType=output  PseudoPeriodic=off  Frequencies=[]  VectorFormat=1-D array  Unit=inherit  AffineConversion=off
  LEy : nesl_utility/PS-Simulink Converter  PhysicalDomain=network_engine_domain  SubClassName=ps_output  LeftPortType=input  RightPortType=output  PseudoPeriodic=off  Frequencies=[]  VectorFormat=1-D array  Unit=inherit  AffineConversion=off
  LEz : nesl_utility/PS-Simulink Converter  PhysicalDomain=network_engine_domain  SubClassName=ps_output  LeftPortType=input  RightPortType=output  PseudoPeriodic=off  Frequencies=[]  VectorFormat=1-D array  Unit=inherit  AffineConversion=off
  LForearmonLArmFGlobal : Gain  Gain=-1
  LForearmonLArmTGlobal : Gain  Gain=-1
  RotationMatrix : nesl_utility/PS-Simulink Converter  PhysicalDomain=network_engine_domain  SubClassName=ps_output  LeftPortType=input  RightPortType=output  PseudoPeriodic=off  Frequencies=[]  VectorFormat=1-D array  Unit=inherit  AffineConversion=off
  Spherical Solid : sm_lib/Body Elements/Spherical Solid  SphereRadius=1.75  SphereRadiusUnits=in  ExportEntireGeometry=off  InertiaType=CalculateFromGeometry  BasedOnType=Density  Density=0  DensityUnits=kg/m^3  Mass=1  MassUnits=kg  CenterOfMass=[0 0 0]  CenterOfMassUnits=m  MomentsOfInertia=[1 1 1]  MomentsOfInertiaUnits=kg*m^2  ProductsOfInertia=[0 0 0]  ProductsOfInertiaUnits=kg*m^2  GraphicType=FromGeometry  MarkerShape=Sphere  MarkerSize=10  GraphicVisPropType=SimpleVisualProperties  GraphicDiffuseColor=[1.0 0.8 0.4]  GraphicOpacity=1  GraphicSpecularColor=[0.5 0.5 0.5 1.0]  GraphicAmbientColor=[0.15 0.15 0.15 1.0]  GraphicEmissiveColor=[0.0 0.0 0.0 1.0]  GraphicShininess=75  DoExposeReferenceFrame=on  SerializedFrames=<Frames/>
  Transform Sensor : sm_lib/Frames and Transforms/Transform Sensor  MeasurementFrame=World  RotationSequence=XYX  SenseAngle=off  SenseAxis=off  SenseQ=off  SenseR=on  SenseRotationSequence=off  SenseOmegaX=off  SenseOmegaY=off  SenseOmegaZ=off  SenseOmega=off  SenseQDot=off  SenseRDot=off  SenseRotationSequenceDot=off  SenseAlphaX=off  SenseAlphaY=off  SenseAlphaZ=off  SenseAlpha=off  SenseQDDot=off  SenseRDDot=off  SenseX=on  SenseY=on  SenseZ=on  SenseXYZ=off  SenseRad=off  SenseAzim=off  SenseDist=off  SenseInc=off  SenseXDot=off  SenseYDot=off  SenseZDot=off  SenseXYZDot=off  SenseRadDot=off  SenseAzimDot=off  SenseDistDot=off  SenseIncDot=off  SenseXDDot=off  SenseYDDot=off  SenseZDDot=off  SenseXYZDDot=off  SenseRadDDot=off  SenseAzimDDot=off  SenseDistDDot=off  SenseIncDDot=off
  Transform Sensor1 : sm_lib/Frames and Transforms/Transform Sensor  MeasurementFrame=World  RotationSequence=XYX  SenseAngle=off  SenseAxis=off  SenseQ=off  SenseR=off  SenseRotationSequence=off  SenseOmegaX=off  SenseOmegaY=off  SenseOmegaZ=off  SenseOmega=on  SenseQDot=off  SenseRDot=off  SenseRotationSequenceDot=off  SenseAlphaX=off  SenseAlphaY=off  SenseAlphaZ=off  SenseAlpha=off  SenseQDDot=off  SenseRDDot=off  SenseX=on  SenseY=on  SenseZ=on  SenseXYZ=off  SenseRad=off  SenseAzim=off  SenseDist=off  SenseInc=off  SenseXDot=off  SenseYDot=off  SenseZDot=off  SenseXYZDot=on  SenseRadDot=off  SenseAzimDot=off  SenseDistDot=off  SenseIncDot=off  SenseXDDot=off  SenseYDDot=off  SenseZDDot=off  SenseXYZDDot=off  SenseRadDDot=off  SenseAzimDDot=off  SenseDistDDot=off  SenseIncDDot=off
  Vector Concatenate : Concatenate  NumInputs=3
  World Frame : sm_lib/Frames and Transforms/World Frame
  Bottom of Left Arm : PMIOPort  Side=Left
  Top of Left Forearm : PMIOPort  Port=2  Side=Right
  tag scope: LArmonLForearmFGlobalOut=global, LArmonLForearmTGlobalOut=global, LEGlobalPosition=global, LForearmonLArmFGlobalOut=global, LForearmonLArmTGlobalOut=global
  wires:
  LArmonLForearmTLocal/1 -> LArmonLForearmTGlobal/2
  LForearmonLArmTGlobal/1 -> [LForearmonLArmTGlobalOut]  "LForearmonLArmTGlobal"
  RotationMatrix/1 -> LArmonLForearmFGlobal/1, LArmonLForearmTGlobal/1
  LArmonLForearmFLocal/1 -> LArmonLForearmFGlobal/2
  LForearmonLArmFGlobal/1 -> [LForearmonLArmFGlobalOut]  "LForearmonLArmFGlobal"
  LArmonLForearmTGlobal/1 -> [LArmonLForearmTGlobalOut], LForearmonLArmTGlobal/1, Dot Product3/1  "LArmonLForearmTGlobal"
  LEgx/1 -> Vector Concatenate/1
  LEgz/1 -> Vector Concatenate/3
  Vector Concatenate/1 -> [LEGlobalPosition]  "LEGlobalPosition"
  LEgy/1 -> Vector Concatenate/2
  Dot Product3/1 -> LEAngularWorkonForearm/1  "LEonForearmAngularPower"
  Dot Product1/1 -> LELinearWorkonForearm/1  "LEonForearmLinearPower"
  LArmonLForearmFGlobal/1 -> [LArmonLForearmFGlobalOut], LForearmonLArmFGlobal/1, LELinearImpulseonForearm/1, Dot Product1/1  "LArmonLForearmFGlobal"
  LEvGlobal/1 -> Dot Product1/2  "LEVGlobal"
  LEAV/1 -> Dot Product3/2  "LEAVGlobal"
  connections:
  Bottom of Left Arm/RConn1 -- Transform Sensor1/RConn1 -- LE Kinematically Driven/LConn1 -- Spherical Solid/RConn1 -- LE Kinetically Driven/LConn1
  World Frame/RConn1 -- Transform Sensor1/LConn1 -- Transform Sensor/LConn1
  RotationMatrix/LConn1 -- Transform Sensor/RConn2
  LEgx/LConn1 -- Transform Sensor/RConn3
  Transform Sensor/RConn5 -- LEgz/LConn1
  LEgy/LConn1 -- Transform Sensor/RConn4
  LEAV/LConn1 -- Transform Sensor1/RConn2
  LEvGlobal/LConn1 -- Transform Sensor1/RConn6
  LEz/LConn1 -- Transform Sensor1/RConn5
  LEy/LConn1 -- Transform Sensor1/RConn4
  LEx/LConn1 -- Transform Sensor1/RConn3
  Top of Left Forearm/RConn1 -- Transform Sensor/RConn1 -- LE Kinematically Driven/RConn1 -- LE Kinetically Driven/RConn1
  LArmonLForearmFLocal/LConn1 -- LE Kinetically Driven/RConn2
  LArmonLForearmTLocal/LConn1 -- LE Kinetically Driven/RConn3

== system ModelCurrentState/Left Forearm ==
  Left Forearm : Subsystem
  Left Forearm MOF : Subsystem  Commented=on
  Left Elbow : PMIOPort  Side=Left
  Left Wrist : PMIOPort  Port=2  Side=Right
  connections:
  Left Forearm/LConn1 -- Left Elbow/RConn1 -- Left Forearm MOF/LConn1
  Left Forearm/RConn1 -- Left Wrist/RConn1

== system ModelCurrentState/Left Hand ==
  BX : nesl_utility/PS-Simulink Converter  PhysicalDomain=network_engine_domain  SubClassName=ps_output  LeftPortType=input  RightPortType=output  PseudoPeriodic=off  Frequencies=[]  VectorFormat=1-D array  Unit=inherit  AffineConversion=off
  BY : nesl_utility/PS-Simulink Converter  PhysicalDomain=network_engine_domain  SubClassName=ps_output  LeftPortType=input  RightPortType=output  PseudoPeriodic=off  Frequencies=[]  VectorFormat=1-D array  Unit=inherit  AffineConversion=off
  BZ : nesl_utility/PS-Simulink Converter  PhysicalDomain=network_engine_domain  SubClassName=ps_output  LeftPortType=input  RightPortType=output  PseudoPeriodic=off  Frequencies=[]  VectorFormat=1-D array  Unit=inherit  AffineConversion=off
  LHRVector : Sum  Inputs=+-
  LHvx : nesl_utility/PS-Simulink Converter  PhysicalDomain=network_engine_domain  SubClassName=ps_output  LeftPortType=input  RightPortType=output  PseudoPeriodic=off  Frequencies=[]  VectorFormat=1-D array  Unit=inherit  AffineConversion=off
  LHvy : nesl_utility/PS-Simulink Converter  PhysicalDomain=network_engine_domain  SubClassName=ps_output  LeftPortType=input  RightPortType=output  PseudoPeriodic=off  Frequencies=[]  VectorFormat=1-D array  Unit=inherit  AffineConversion=off
  LHvz : nesl_utility/PS-Simulink Converter  PhysicalDomain=network_engine_domain  SubClassName=ps_output  LeftPortType=input  RightPortType=output  PseudoPeriodic=off  Frequencies=[]  VectorFormat=1-D array  Unit=inherit  AffineConversion=off
  LHx : nesl_utility/PS-Simulink Converter  PhysicalDomain=network_engine_domain  SubClassName=ps_output  LeftPortType=input  RightPortType=output  PseudoPeriodic=off  Frequencies=[]  VectorFormat=1-D array  Unit=inherit  AffineConversion=off
  LHy : nesl_utility/PS-Simulink Converter  PhysicalDomain=network_engine_domain  SubClassName=ps_output  LeftPortType=input  RightPortType=output  PseudoPeriodic=off  Frequencies=[]  VectorFormat=1-D array  Unit=inherit  AffineConversion=off
  LHz : nesl_utility/PS-Simulink Converter  PhysicalDomain=network_engine_domain  SubClassName=ps_output  LeftPortType=input  RightPortType=output  PseudoPeriodic=off  Frequencies=[]  VectorFormat=1-D array  Unit=inherit  AffineConversion=off
  LW Unit Vector : MATLAB Function  TreatAsAtomicUnit=on  SystemSampleTime=0
  LWAV : nesl_utility/PS-Simulink Converter  PhysicalDomain=network_engine_domain  SubClassName=ps_output  LeftPortType=input  RightPortType=output  PseudoPeriodic=off  Frequencies=[]  VectorFormat=1-D array  Unit=deg/s  AffineConversion=off
  LeftHandPath UnitVector : Mux  Inputs=3
  Mux1 : Mux  Inputs=3
  Mux2 : Mux  Inputs=3
  Mux8 : Mux  Inputs=3
  Transform Sensor6 : sm_lib/Frames and Transforms/Transform Sensor  MeasurementFrame=World  RotationSequence=XYX  SenseAngle=off  SenseAxis=off  SenseQ=off  SenseR=off  SenseRotationSequence=off  SenseOmegaX=off  SenseOmegaY=off  SenseOmegaZ=off  SenseOmega=off  SenseQDot=off  SenseRDot=off  SenseRotationSequenceDot=off  SenseAlphaX=off  SenseAlphaY=off  SenseAlphaZ=off  SenseAlpha=off  SenseQDDot=off  SenseRDDot=off  SenseX=on  SenseY=on  SenseZ=on  SenseXYZ=off  SenseRad=off  SenseAzim=off  SenseDist=off  SenseInc=off  SenseXDot=off  SenseYDot=off  SenseZDot=off  SenseXYZDot=off  SenseRadDot=off  SenseAzimDot=off  SenseDistDot=off  SenseIncDot=off  SenseXDDot=off  SenseYDDot=off  SenseZDDot=off  SenseXYZDDot=off  SenseRadDDot=off  SenseAzimDDot=off  SenseDistDDot=off  SenseIncDDot=off
  Transform Sensor7 : sm_lib/Frames and Transforms/Transform Sensor  MeasurementFrame=World  RotationSequence=XYX  SenseAngle=off  SenseAxis=off  SenseQ=off  SenseR=off  SenseRotationSequence=off  SenseOmegaX=off  SenseOmegaY=off  SenseOmegaZ=off  SenseOmega=on  SenseQDot=off  SenseRDot=off  SenseRotationSequenceDot=off  SenseAlphaX=off  SenseAlphaY=off  SenseAlphaZ=off  SenseAlpha=off  SenseQDDot=off  SenseRDDot=off  SenseX=on  SenseY=on  SenseZ=on  SenseXYZ=off  SenseRad=off  SenseAzim=off  SenseDist=off  SenseInc=off  SenseXDot=on  SenseYDot=on  SenseZDot=on  SenseXYZDot=off  SenseRadDot=off  SenseAzimDot=off  SenseDistDot=off  SenseIncDot=off  SenseXDDot=off  SenseYDDot=off  SenseZDDot=off  SenseXYZDDot=off  SenseRadDDot=off  SenseAzimDDot=off  SenseDistDDot=off  SenseIncDDot=off
  Butt : PMIOPort  Side=Right
  Global Reference : PMIOPort  Port=2  Side=Right
  LH : PMIOPort  Port=3  Side=Right
  tag scope: LHAVGlobal=global, LHPathUV=global, LHRVector=global, LHVGlobal=global
  wires:
  LW Unit Vector/3(LWuvy) -> LeftHandPath UnitVector/2
  LHRVector/1 -> [LHRVector]
  LHx/1 -> Mux2/1  "LHx"
  LHvy/1 -> LW Unit Vector/3(LWvy), Mux8/2, Mux1/2  "LHvy"
  LW Unit Vector/4(LWuvz) -> LeftHandPath UnitVector/3
  LW Unit Vector/2(LWuvx) -> LeftHandPath UnitVector/1
  Mux1/1 -> [LHVGlobal]  "LHVGlobal"
  LHvz/1 -> Mux1/3, LW Unit Vector/4(LWvz), Mux8/3  "LHvz"
  LHvx/1 -> Mux1/1, LW Unit Vector/2(LWvx), Mux8/1  "LHvx"
  Mux8/1 -> LW Unit Vector/1(LWv)
  LHy/1 -> Mux2/2  "LHy"
  LHz/1 -> Mux2/3  "LHz"
  LWAV/1 -> [LHAVGlobal]  "LHAVGlobal"
  Mux2/1 -> LHRVector/1  "LeftHandPostion"
  LeftHandPath UnitVector/1 -> [LHPathUV]  "LHPathUV"
  [ClubCOM] -> LHRVector/2
  connections:
  Global Reference/RConn1 -- Transform Sensor6/LConn1 -- Transform Sensor7/LConn1
  BX/LConn1 -- Transform Sensor6/RConn2
  LWAV/LConn1 -- Transform Sensor7/RConn2
  LHx/LConn1 -- Transform Sensor7/RConn3
  LHy/LConn1 -- Transform Sensor7/RConn4
  Butt/RConn1 -- Transform Sensor6/RConn1
  LHvz/LConn1 -- Transform Sensor7/RConn8
  LHvx/LConn1 -- Transform Sensor7/RConn6
  LHz/LConn1 -- Transform Sensor7/RConn5
  BY/LConn1 -- Transform Sensor6/RConn3
  BZ/LConn1 -- Transform Sensor6/RConn4
  LHvy/LConn1 -- Transform Sensor7/RConn7
  Transform Sensor7/RConn1 -- LH/RConn1

== system ModelCurrentState/Left Scapula Joint ==
  LScap Kinematically Driven : Subsystem  Commented=on
  LScap Kinetically Driven : Subsystem
  COM Rod Top : PMIOPort  Side=Left
  Hub : PMIOPort  Port=2  Side=Right
  connections:
  COM Rod Top/RConn1 -- LScap Kinetically Driven/LConn1 -- LScap Kinematically Driven/LConn1
  Hub/RConn1 -- LScap Kinematically Driven/RConn1 -- LScap Kinetically Driven/RConn1
